simulink model "Simulink_Ex4"  (R2024b)
settings: Solver=VariableStepAuto  StartTime=0.0  StopTime=100.0  RelTol=1e-3
values from neighbouring files (symbols this model uses):
  x0 = 1    [Ex4_sccript.m]
settings Model: Creator=eduardo  LastModifiedBy=eduardo
settings DataIOCC: SaveFormat=Array  ReturnWorkspaceOutputs=off

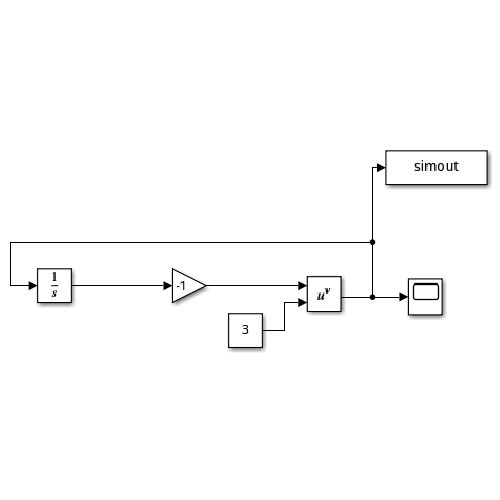
[thumbnail: Simulink's stored preview of the top-level diagram]
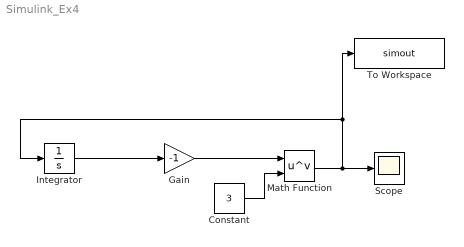
== system Simulink_Ex4 ==
  Constant : Constant  Value=3
  Gain : Gain  Gain=-1
  Integrator : Integrator  InitialCondition=x0
  Math Function : Math  Operator=pow  OutputSignalType=real
  Scope : Scope
  To Workspace : ToWorkspace  VariableName=simout  SampleTime=-1
  wires:
  Integrator/1 -> Gain/1
  Gain/1 -> Math Function/1
  Constant/1 -> Math Function/2
  Math Function/1 -> Scope/1, To Workspace/1, Integrator/1
